simulink model "Requirements_Table"  (R2022a)
settings: Solver=FixedStepAuto  StartTime=0.0  StopTime=10  FixedStep=1e-3  RelTol=1e-3  EnableMultiTasking=on
undefined symbols (not defined in the file): D0, D1, D10, D11, D12, D13, D2, D3, D4, D5, D6, D7, D8, D9, PTA0, PTA1, PTA2, PTB23, PTB9, PTC16, PTC17, PTC2, PTC3, PTC4, PTD0, PTD1, PTD2, PTD3
libraries: frdmk64flib x16
settings Model: ExtModeTrigDuration=5  Creator=pauls  LastModifiedBy=young
settings OptimizationCC: EnhancedBackFolding=on  PassReuseOutputArgsAs=Individual arguments  ZeroExternalMemoryAtStartup=off  ZeroInternalMemoryAtStartup=off  MaxStackSize=64  OptimizeBlockOrder=speed  DifferentSizesBufferReuse=on  OptimizationCustomize=off  EfficientTunableParamExpr=on
settings DebuggingCC: ParameterTunabilityLossMsg=error
settings HardwareCC: ProdBitPerPointer=32  ProdBitPerSizeT=32  ProdBitPerPtrDiffT=32  ProdLargestAtomicInteger=Long  ProdLargestAtomicFloat=Double  ProdWordSize=32  ProdHWDeviceType=ARM Compatible->ARM Cortex
settings SFSimCC: MATLABDynamicMemAlloc=off
settings RTWCC: SystemTargetFile=ert.tlc  HardwareBoard=NXP FRDM-K64F  TLCOptions="-aInlineSetEventsForThisBaseRateFcn=TLC_FALSE -aSuppressMultiTaskScheduler=TLC_FALSE  -aRateBasedStepFcn=0"  TemplateMakefile=ert_default_tmf  Toolchain=GNU Tools for ARM Embedded Processors
settings CodeAppCC: ForceParamTrailComments=on  IgnoreCustomStorageClasses=off  OperatorAnnotations=on  SimulinkDataObjDesc=on  SFDataObjDesc=on  InsertBlockDesc=on
settings ERTTargetCC: ExtModeTransport=4  ExtModeMexFile=sendToCommService

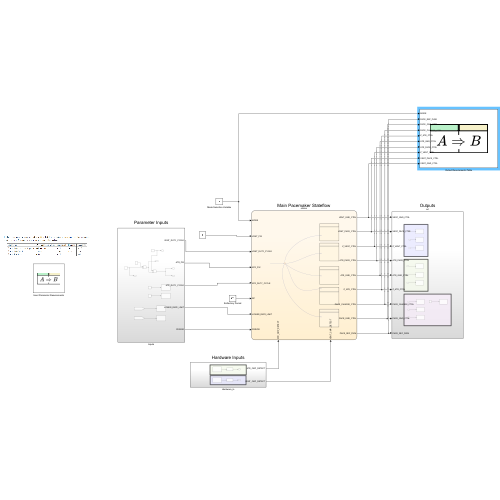
[thumbnail: Simulink's stored preview of the top-level diagram]
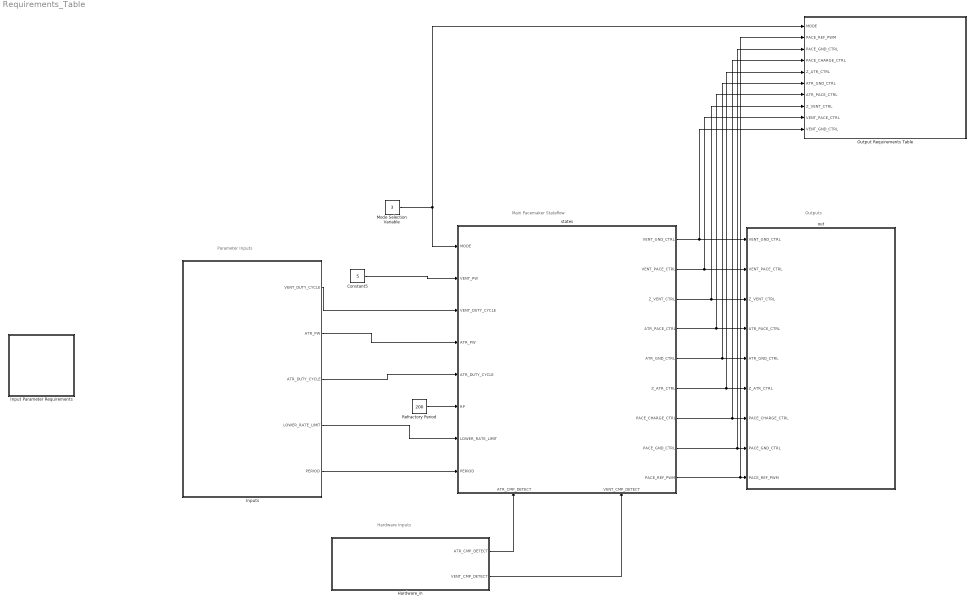
== system Requirements_Table ==
  note: Main Pacemaker Stateflow
  note: Outputs
  note: Hardware Inputs
  note: Parameter Inputs
  " states  " : Stateflow chart  TreatAsAtomicUnit=on
      settings: PortSchema="{\"entries\":[{\"content\":{\"sides\":[{\"content\":{\"connectorIds\":[\"In1\",\"In4\",\"In5\",\"In7\",\"In6\",\"In9\",\"In10\",\"In8\"]},\"type\":\"ConnectorPlacement.EquallySpacedRectSide\",\"uuid\":\"01118a3a-35ab-415d-a4dc-7a9e5022dc58\"},{\"content\":{\"connectorIds\":[\"Out1\",\"Out2\",\"Out3\",\"Out4\",\"Out5\",\"Out6\",\"Out7\",\"Out8\",\"Out9\"],\"side\":\"RIGHT\"},\"type\":\"ConnectorPlacement.EquallySpacedRectSide\",\"uuid\":\"d119b6db-c579-45b6-8580-2a3960ab3129\"},{\"content\":{\"connectorIds\":[],\"side\":\"TOP\"},\"type\":\"ConnectorPlacement.EquallySpacedRectSide\",\"uuid\":\"18fa5379-1691-4053-811b-8d647a346445\"},{\"content\":{\"connectorIds\":[\"In2\",\"In3\"],\"side\":\"BOTTOM\"},\"type\":\"ConnectorPlacement.EquallySpacedRectSide\",\"uuid\":\"c19ca9f7-b829-4e11-b03e-3e9d42b35795\"}]},\"type\":\"ConnectorPlacement.EquallySpacedConnector\",\"uuid\":\"6e6fa963-33ea-4c14-97b4-73e5587667a9\"}],\"packageUris\":[\"http://schema.mathworks.com/mf0/Connector/R2020b\"],\"version\":\"1.0\"}"
  Constant5 : Constant  Value=5
  Hardware_in : Subsystem
  Input Parameter Requirements : Requirements Table  TreatAsAtomicUnit=on
  Inputs : Subsystem
  Mode Selection Variable : Constant  Value=3
  Output Requirements Table : Requirements Table  TreatAsAtomicUnit=on
  Refractory Period : Constant  Value=200
  "out " : Subsystem
  wires:
  " states  "/7(PACE_CHARGE_CTRL) -> Output Requirements Table/4(PACE_CHARGE_CTRL), "out "/7(PACE_CHARGE_CTRL)
  Inputs/5(PERIOD) -> " states  "/8(PERIOD)
  " states  "/5(ATR_GND_CTRL) -> Output Requirements Table/6(ATR_GND_CTRL), "out "/5(ATR_GND_CTRL)
  Constant5/1 -> " states  "/4(VENT_PW)
  " states  "/2(VENT_PACE_CTRL) -> Output Requirements Table/9(VENT_PACE_CTRL), "out "/2(VENT_PACE_CTRL)
  Inputs/4(LOWER_RATE_LIMIT) -> " states  "/10(LOWER_RATE_LIMIT)
  " states  "/6(Z_ATR_CTRL) -> Output Requirements Table/5(Z_ATR_CTRL), "out "/6(Z_ATR_CTRL)
  " states  "/3(Z_VENT_CTRL) -> Output Requirements Table/8(Z_VENT_CTRL), "out "/3(Z_VENT_CTRL)
  " states  "/8(PACE_GND_CTRL) -> Output Requirements Table/3(PACE_GND_CTRL), "out "/8(PACE_GND_CTRL)
  Inputs/1(VENT_DUTY_CYCLE) -> " states  "/5(VENT_DUTY_CYCLE)
  Refractory Period/1 -> " states  "/9(RP)
  " states  "/4(ATR_PACE_CTRL) -> Output Requirements Table/7(ATR_PACE_CTRL), "out "/4(ATR_PACE_CTRL)
  Inputs/3(ATR_DUTY_CYCLE) -> " states  "/6(ATR_DUTY_CYCLE)
  " states  "/9(PACE_REF_PWM) -> Output Requirements Table/2(PACE_REF_PWM), "out "/9(PACE_REF_PWM)
  Hardware_in/2(VENT_CMP_DETECT) -> " states  "/3(VENT_CMP_DETECT)
  " states  "/1(VENT_GND_CTRL) -> Output Requirements Table/10(VENT_GND_CTRL), "out "/1(VENT_GND_CTRL)
  Inputs/2(ATR_PW) -> " states  "/7(ATR_PW)
  Mode Selection Variable/1 -> " states  "/1(MODE), Output Requirements Table/1(MODE)
  Hardware_in/1(ATR_CMP_DETECT) -> " states  "/2(ATR_CMP_DETECT)

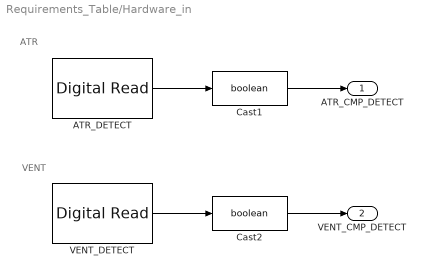
== system Requirements_Table/Hardware_in ==
  note: VENT
  note: ATR
  ATR_DETECT : frdmk64flib/Digital Read  Whichpin=PTC16 (D0)  SampleTime=-1
  Cast1 : DataTypeConversion  OutDataTypeStr=boolean  SaturateOnIntegerOverflow=off  RndMeth=Floor
  Cast2 : DataTypeConversion  OutDataTypeStr=boolean  SaturateOnIntegerOverflow=off  RndMeth=Floor
  VENT_DETECT : frdmk64flib/Digital Read  Whichpin=PTC17 (D1)  SampleTime=-1
  ATR_CMP_DETECT : Outport
  VENT_CMP_DETECT : Outport  Port=2
  wires:
  Cast1/1 -> ATR_CMP_DETECT/1
  ATR_DETECT/1 -> Cast1/1
  VENT_DETECT/1 -> Cast2/1
  Cast2/1 -> VENT_CMP_DETECT/1

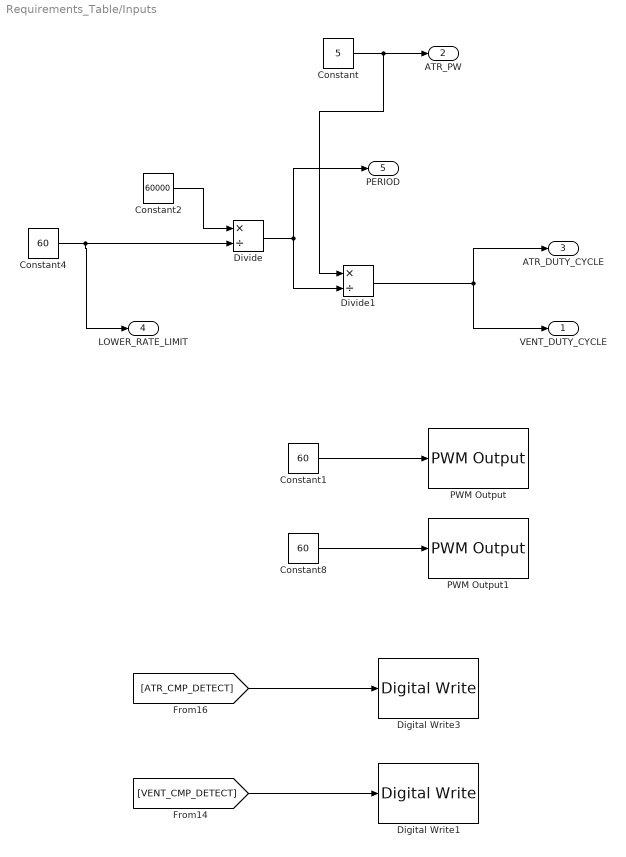
== system Requirements_Table/Inputs ==
  Constant : Constant  Value=5
  Constant1 : Constant  Value=60
  Constant2 : Constant  Value=60000
  Constant4 : Constant  Value=60
  Constant8 : Constant  Value=60
  Digital Write1 : frdmk64flib/Digital Write  Whichpin=GREEN_LED
  Digital Write3 : frdmk64flib/Digital Write  Whichpin=BLUE_LED
  Divide : Product  Inputs=*/
  Divide1 : Product  Inputs=*/
  PWM Output : frdmk64flib/PWM Output  Whichpin=PTA1 (D3)  InitialFrequency=2000  InitialDutyCycle=0
  PWM Output1 : frdmk64flib/PWM Output  Whichpin=PTC2 (D6)  InitialFrequency=2000  InitialDutyCycle=0
  VENT_DUTY_CYCLE : Outport
  ATR_PW : Outport  Port=2
  ATR_DUTY_CYCLE : Outport  Port=3
  LOWER_RATE_LIMIT : Outport  Port=4
  PERIOD : Outport  Port=5
  wires:
  Constant/1 -> ATR_PW/1, Divide1/1
  Constant4/1 -> LOWER_RATE_LIMIT/1, Divide/2
  Divide/1 -> PERIOD/1, Divide1/2
  Divide1/1 -> VENT_DUTY_CYCLE/1, ATR_DUTY_CYCLE/1
  Constant2/1 -> Divide/1
  [VENT_CMP_DETECT] -> Digital Write1/1
  Constant8/1 -> PWM Output1/1
  Constant1/1 -> PWM Output/1
  [ATR_CMP_DETECT] -> Digital Write3/1

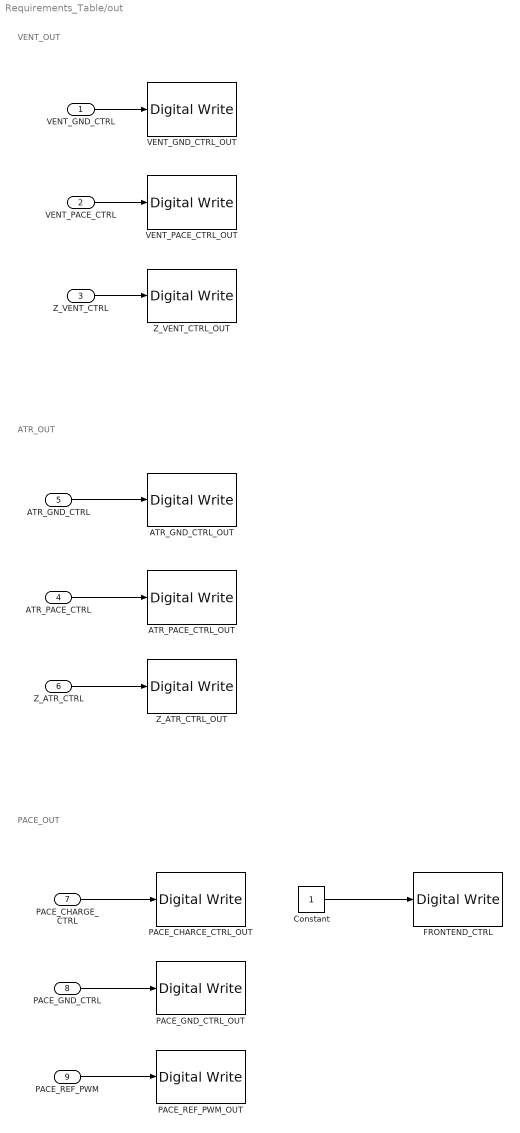
== system Requirements_Table/out  ==
  note: PACE_OUT
  note: ATR_OUT
  note: VENT_OUT
  VENT_GND_CTRL : Inport
  VENT_PACE_CTRL : Inport  Port=2
  Z_VENT_CTRL : Inport  Port=3
  ATR_PACE_CTRL : Inport  Port=4
  ATR_GND_CTRL : Inport  Port=5
  Z_ATR_CTRL : Inport  Port=6
  PACE_CHARGE_CTRL : Inport  Port=7
  PACE_GND_CTRL : Inport  Port=8
  PACE_REF_PWM : Inport  Port=9
  ATR_GND_CTRL_OUT : frdmk64flib/Digital Write  Whichpin=PTD2 (D11)
  ATR_PACE_CTRL_OUT : frdmk64flib/Digital Write  Whichpin=PTA0 (D8)
  Constant : Constant
  FRONTEND_CTRL : frdmk64flib/Digital Write  Whichpin=PTD1 (D13)
  PACE_CHARCE_CTRL_OUT : frdmk64flib/Digital Write  Whichpin=PTB9 (D2)
  PACE_GND_CTRL_OUT : frdmk64flib/Digital Write  Whichpin=PTD0 (D10)
  PACE_REF_PWM_OUT : frdmk64flib/Digital Write  Whichpin=PTA2 (D5)
  VENT_GND_CTRL_OUT : frdmk64flib/Digital Write  Whichpin=PTD3 (D12)
  VENT_PACE_CTRL_OUT : frdmk64flib/Digital Write  Whichpin=PTC4 (D9)
  Z_ATR_CTRL_OUT : frdmk64flib/Digital Write  Whichpin=PTB23 (D4)
  Z_VENT_CTRL_OUT : frdmk64flib/Digital Write  Whichpin=PTC3 (D7)
  wires:
  VENT_GND_CTRL/1 -> VENT_GND_CTRL_OUT/1
  VENT_PACE_CTRL/1 -> VENT_PACE_CTRL_OUT/1
  Z_VENT_CTRL/1 -> Z_VENT_CTRL_OUT/1
  ATR_GND_CTRL/1 -> ATR_GND_CTRL_OUT/1
  Z_ATR_CTRL/1 -> Z_ATR_CTRL_OUT/1
  ATR_PACE_CTRL/1 -> ATR_PACE_CTRL_OUT/1
  PACE_CHARGE_CTRL/1 -> PACE_CHARCE_CTRL_OUT/1
  PACE_REF_PWM/1 -> PACE_REF_PWM_OUT/1
  PACE_GND_CTRL/1 -> PACE_GND_CTRL_OUT/1
  Constant/1 -> FRONTEND_CTRL/1

== stateflow chart Requirements_Table/Input Parameter Requirements ==
  (default) -> (junction 1073741930)
  (junction 1073741930) -> (junction 1073741931) : {
      | % SF_REQ_REV_07
      | }
  (junction 1073741931) -> (junction 1073741933) : {
      | % HEADER_ASSIGNMENTS
      |
      | }
  (junction 1073741933) -> (junction 1073741935) : {
      | % START_A_4
      | }
  (junction 1073741935) -> (junction 1073741937) : {
      | }
  (junction 1073741937) -> (junction 1073741939)
  (junction 1073741939) -> (junction 1073741941) : {
      | }
  (junction 1073741941) -> (junction 1073741943) : {
      | % END_A_4
      | }
  (junction 1073741943) -> (junction 1073741945) : {
      | % START_R_1
      | }
  (junction 1073741945) -> (junction 1073741947) : {
      | }
  (junction 1073741947) -> (junction 1073741949)
  (junction 1073741949) -> (junction 1073741951) [order 1] : [(((p_aPaceAmp) == (0 || [0.112, 5.6]))) && (((p_vPaceAmp) == (0 || [0.112, 5.6]))) && (((p_aPaceWidth) >= (1) && (p_aPaceWidth) <= (31))) && (((p_vPaceWidth) >= (1) && (p_vPaceWidth) <= (31))) && (((p_aSensitivity) >= (0) && (p_aSensitivity) <= (5))) && (((p_vSensitivity) >= (0) && (p_vSensitivity) <= (5))) && ([150,500] && p_aPaceWidth < (p_ARP)< p_lowrateInterval) && ([150,500] && p_vPaceWidth < (p_VRP) < p_lowrateInterval) && (((p_lowrateInterval ) >= (343) && (p_lowrateInterval ) <= (2000))) && (((p_pacingMode ) == (1)) || ((p_pacingMode ) == (2)) || ((p_pacingMode ) == (3)) || ((p_pacingMode ) == (4)) || ((p_pacingMode ) == (5)))]
  (junction 1073741949) -> (junction 1073741957) [order 2]
  (junction 1073741951) -> (junction 1073741953) : {
      | Pass
      |
      | }
  (junction 1073741953) -> (junction 1073741955) : {
      | }
  (junction 1073741955) -> (junction 1073741957)
  (junction 1073741957) -> (junction 1073741959)
  (junction 1073741959) -> (junction 1073741961) : {
      | % END_R_1
      | }

== stateflow chart Requirements_Table/Output Requirements Table ==
  (default) -> (junction 1073744155)
  (junction 1073744155) -> (junction 1073744156) : {
      | % SF_REQ_REV_07
      | }
  (junction 1073744156) -> (junction 1073744158) : {
      | % HEADER_ASSIGNMENTS
      |
      | }
  (junction 1073744158) -> (junction 1073744160) : {
      | % START_A_4
      | }
  (junction 1073744160) -> (junction 1073744162) : {
      | }
  (junction 1073744162) -> (junction 1073744164)
  (junction 1073744164) -> (junction 1073744166) : {
      | }
  (junction 1073744166) -> (junction 1073744168) : {
      | % END_A_4
      | }
  (junction 1073744168) -> (junction 1073744170) : {
      | % START_R_1
      | }
  (junction 1073744170) -> (junction 1073744172) : {
      | }
  (junction 1073744172) -> (junction 1073744174)
  (junction 1073744174) -> (junction 1073744176) [order 1] : [(((MODE) == (1)) || ((MODE) == (4))) && (((ATR_GND_CTRL) == (True))) && (((ATR_PACE_CTRL) == (False))) && (((VENT_GND_CTRL) == (False))) && (((VENT_PACE_CTRL) == (False))) && (((PACE_CHARGE_CTRL) == (True))) && (((PACE_GND_CTRL) == (False)))]
  (junction 1073744174) -> (junction 1073744182) [order 2]
  (junction 1073744176) -> (junction 1073744178) : {
      | reqtable_postcondition((((ATR_GND_CTRL) == (False))) && (((ATR_PACE_CTRL) == (True))) && (((VENT_GND_CTRL) == (High))) && (((VENT_PACE_CTRL) == (False))) && (((PACE_GND_CTRL) == (True))), 'R:1');
      |
      |
      | }
  (junction 1073744178) -> (junction 1073744180) : {
      | }
  (junction 1073744180) -> (junction 1073744182)
  (junction 1073744182) -> (junction 1073744184)
  (junction 1073744184) -> (junction 1073744186) : {
      | % END_R_1
      | }
  (junction 1073744186) -> (junction 1073744188) : {
      | % START_R_7
      | }
  (junction 1073744188) -> (junction 1073744190) : {
      | }
  (junction 1073744190) -> (junction 1073744192)
  (junction 1073744192) -> (junction 1073744194) [order 1] : [(((MODE) == (1)) || ((MODE) == (4)))]
  (junction 1073744192) -> (junction 1073744200) [order 2]
  (junction 1073744194) -> (junction 1073744196) : {
      |
      |
      | }
  (junction 1073744196) -> (junction 1073744198) : {
      | }
  (junction 1073744198) -> (junction 1073744200)
  (junction 1073744200) -> (junction 1073744202)
  (junction 1073744202) -> (junction 1073744204) : {
      | % END_R_7
      | }
  (junction 1073744204) -> (junction 1073744206) : {
      | % START_R_10
      | }
  (junction 1073744206) -> (junction 1073744208) : {
      | }
  (junction 1073744208) -> (junction 1073744210)
  (junction 1073744210) -> (junction 1073744212) [order 1] : [(((MODE) == (2)) || ((MODE) == (3))) && (((ATR_GND_CTRL) == (False))) && (((ATR_PACE_CTRL) == (False))) && (((VENT_GND_CTRL) == (True))) && (((VENT_PACE_CTRL) == (False)))]
  (junction 1073744210) -> (junction 1073744218) [order 2]
  (junction 1073744212) -> (junction 1073744214) : {
      |
      |
      | }
  (junction 1073744214) -> (junction 1073744216) : {
      | }
  (junction 1073744216) -> (junction 1073744218)
  (junction 1073744218) -> (junction 1073744220)
  (junction 1073744220) -> (junction 1073744222) : {
      | % END_R_10
      | }
  (junction 1073744222) -> (junction 1073744224) : {
      | % START_R_13
      | }
  (junction 1073744224) -> (junction 1073744226) : {
      | }
  (junction 1073744226) -> (junction 1073744228)
  (junction 1073744228) -> (junction 1073744230) [order 1] : [(((MODE) == (2)) || ((MODE) == (3)))]
  (junction 1073744228) -> (junction 1073744236) [order 2]
  (junction 1073744230) -> (junction 1073744232) : {
      |
      |
      | }
  (junction 1073744232) -> (junction 1073744234) : {
      | }
  (junction 1073744234) -> (junction 1073744236)
  (junction 1073744236) -> (junction 1073744238)
  (junction 1073744238) -> (junction 1073744240) : {
      | % END_R_13
      | }
  data: MODE input; PACE_REF_PWM input; PACE_GND_CTRL input; PACE_CHARGE_CTRL input; Z_ATR_CTRL input; ATR_GND_CTRL input; ATR_PACE_CTRL input; Z_VENT_CTRL input; VENT_PACE_CTRL input; VENT_GND_CTRL input

== stateflow chart Requirements_Table/ states   ==
  state AOO [group]
    state CharingC22
      %Capacitor charing state
      ATR_PACE_CTRL = LOW
      VENT_PACE_CTRL = LOW
      PACE_REF_PWM = ATR_DUTY_CYCLE
      PACE_CHARGE_CTRL = HIGH
      %Discharge capacitor
      PACE_GND_CTRL = HIGH
      VENT_PACE_CTRL = LOW
      Z_ATR_CTRL = LOW
      Z_VENT_CTRL = LOW
      ATR_PACE_CTRL = LOW
      ATR_GND_CTRL = LOW
      VENT_GND_CTRL = HIGH
    state AVPacing
      %step 2
      PACE_CHARGE_CTRL = LOW
      PACE_GND_CTRL = HIGH
      ATR_PACE_CTRL = HIGH
      ATR_GND_CTRL = LOW
      Z_ATR_CTRL = LOW
      Z_VENT_CTRL = LOW
      VENT_GND_CTRL = LOW
      VENT_PACE_CTRL = LOW
    AOO.CharingC22 -> AOO.AVPacing : after(PERIOD-ATR_PW, msec)
    AOO.AVPacing -> AOO.CharingC22 : after(ATR_PW, msec)
  state VOO [group]
    state CharingC23
      during:
      %Begin Charging C22 Capacitor
      ATR_PACE_CTRL = LOW
      VENT_PACE_CTRL = LOW
      PACE_REF_PWM = VENT_DUTY_CYCLE
      PACE_CHARGE_CTRL = HIGH
      %Begin Discharging C21 Blocking Capacitor
      PACE_GND_CTRL = HIGH
      VENT_PACE_CTRL = LOW
      Z_ATR_CTRL = LOW
      Z_VENT_CTRL = LOW
      ATR_PACE_CTRL = LOW
      ATR_GND_CTRL = LOW
      VENT_GND_CTRL = HIGH
    state Discharge
      during:
      %Discharge C22 into Ventricle (Vent Pacing)
      %Begin Charging Blocking Capacitor
      PACE_CHARGE_CTRL = LOW
      PACE_GND_CTRL = HIGH
      ATR_PACE_CTRL = LOW
      ATR_GND_CTRL = LOW
      Z_ATR_CTRL = LOW
      Z_VENT_CTRL = LOW
      VENT_GND_CTRL = LOW
      VENT_PACE_CTRL  = HIGH
    VOO.CharingC23 -> VOO.Discharge : after(PERIOD-VENT_PW, msec)
    VOO.Discharge -> VOO.CharingC23 : after(VENT_PW, msec)
  state VVI [group]
    state CharingC23
      during:
      %Begin Charging C22 Capacitor
      ATR_PACE_CTRL = LOW
      VENT_PACE_CTRL = LOW
      PACE_REF_PWM = VENT_DUTY_CYCLE
      PACE_CHARGE_CTRL = HIGH
      %Begin Discharging C21 Blocking Capacitor
      PACE_GND_CTRL = HIGH
      VENT_PACE_CTRL = LOW
      Z_ATR_CTRL = LOW
      Z_VENT_CTRL = LOW
      ATR_PACE_CTRL = LOW
      ATR_GND_CTRL = LOW
      VENT_GND_CTRL = HIGH
    state Discharge
      during:
      %Discharge C22 into Ventricle (Vent Pacing)
      %Begin Charging Blocking Capacitor
      PACE_CHARGE_CTRL = LOW
      PACE_GND_CTRL = HIGH
      ATR_PACE_CTRL = LOW
      ATR_GND_CTRL = LOW
      Z_ATR_CTRL = LOW
      Z_VENT_CTRL = LOW
      VENT_GND_CTRL = LOW
      VENT_PACE_CTRL  = HIGH
    state Inhibit
      PACE_GND_CTRL = HIGH
      VENT_PACE_CTRL = LOW
      Z_ATR_CTRL = LOW
      Z_VENT_CTRL = LOW
      ATR_PACE_CTRL = LOW
      ATR_GND_CTRL = LOW
      VENT_GND_CTRL = HIGH
    VVI.CharingC23 -> VVI.Discharge [order 1] : after(PERIOD-VENT_PW, msec)[VENT_CMP_DETECT == LOW]
    VVI.CharingC23 -> VVI.Inhibit [order 2] : after(LOWER_RATE_LIMIT, msec)[VENT_CMP_DETECT == HIGH]
    VVI.Inhibit -> VVI.CharingC23 : after(RP,msec)
    VVI.Discharge -> VVI.Inhibit : after(VENT_PW, msec)
  state AAI [group]
    state AVPacing
      %step 2
      PACE_CHARGE_CTRL = LOW
      PACE_GND_CTRL = HIGH
      ATR_PACE_CTRL = HIGH
      ATR_GND_CTRL = LOW
      Z_ATR_CTRL = LOW
      Z_VENT_CTRL = LOW
      VENT_GND_CTRL = LOW
      VENT_PACE_CTRL = LOW
    state CharingC22
      %Capacitor charing state
      ATR_PACE_CTRL = LOW
      VENT_PACE_CTRL = LOW
      PACE_REF_PWM = ATR_DUTY_CYCLE
      PACE_CHARGE_CTRL = HIGH
      %Discharge capacitor
      PACE_GND_CTRL = HIGH
      VENT_PACE_CTRL = LOW
      Z_ATR_CTRL = LOW
      Z_VENT_CTRL = LOW
      ATR_PACE_CTRL = LOW
      ATR_GND_CTRL = LOW
      VENT_GND_CTRL = HIGH
    state Inhibit
      %Through Trial and error found that discharging
      %again will fix the pacing during AAI
      PACE_GND_CTRL = HIGH
      VENT_PACE_CTRL = LOW
      Z_ATR_CTRL = LOW
      Z_VENT_CTRL = LOW
      ATR_PACE_CTRL = LOW
      ATR_GND_CTRL = LOW
      VENT_GND_CTRL = HIGH
    AAI.CharingC22 -> AAI.AVPacing [order 2] : after(PERIOD-ATR_PW, msec)
    AAI.CharingC22 -> AAI.Inhibit [order 1] : after(LOWER_RATE_LIMIT,msec)[ATR_CMP_DETECT == HIGH]
    AAI.AVPacing -> AAI.Inhibit : after(ATR_PW, msec)
    AAI.Inhibit -> AAI.CharingC22 : after(RP,msec)
  state TEST [group]
    state CharingC23
      %Capacitor charing state
      ATR_PACE_CTRL = LOW
      VENT_PACE_CTRL = LOW
      PACE_REF_PWM = ATR_DUTY_CYCLE
      PACE_CHARGE_CTRL = HIGH
      %Discharge capacitor
      PACE_GND_CTRL = HIGH
      VENT_PACE_CTRL = LOW
      Z_ATR_CTRL = LOW
      Z_VENT_CTRL = LOW
      ATR_PACE_CTRL = LOW
      ATR_GND_CTRL = LOW
      VENT_GND_CTRL = HIGH
    state AVPacing1
      %step 2
      PACE_CHARGE_CTRL = LOW
      PACE_GND_CTRL = HIGH
      ATR_PACE_CTRL = HIGH
      ATR_GND_CTRL = LOW
      Z_ATR_CTRL = LOW
      Z_VENT_CTRL = LOW
      VENT_GND_CTRL = LOW
      VENT_PACE_CTRL = LOW
    TEST.CharingC23 -> AVPacing1 : after(PERIOD-ATR_PW, msec)
    AVPacing1 -> TEST.CharingC23 : after(ATR_PW, msec)
  (junction 37) -> TEST.CharingC23 [order 5]
  (junction 37) -> VVI.CharingC23 [order 3] : [MODE ==3]
  (junction 37) -> AAI.CharingC22 [order 4] : [MODE == 4]
  (junction 37) -> AOO.CharingC22 [order 1] : [MODE ==1]
  (junction 37) -> VOO.CharingC23 [order 2] : [MODE ==2]
  (default) -> (junction 37)
  data: MODE input; ATR_CMP_DETECT input; VENT_CMP_DETECT input; VENT_GND_CTRL output; VENT_PACE_CTRL output; Z_VENT_CTRL output; ATR_PACE_CTRL output; VENT_PW input; VENT_DUTY_CYCLE input; HIGH local =true; LOW local =false; ATR_GND_CTRL output; Z_ATR_CTRL output; PACE_CHARGE_CTRL output; PACE_GND_CTRL output; PACE_REF_PWM output; ATR_DUTY_CYCLE input; ATR_PW input; PERIOD input; RP input; LOWER_RATE_LIMIT input
